simulink model "P6"  (R2019a)
settings: Solver=VariableStepAuto  StartTime=0.0  StopTime=20.0  RelTol=1e-3
undefined symbols (not defined in the file): P_reduced
settings Model: Creator=ADMIN  LastModifiedBy=ADMIN

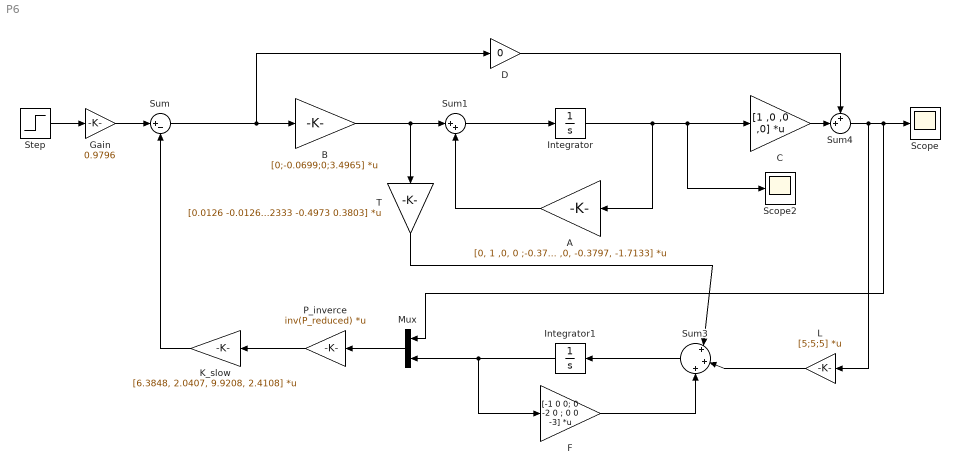
== system P6 ==
  A : Gain  Gain=[0, 1 ,0, 0 ;-0.378 ,0 ,7.0147 ,0.0343;0, 0, 0, 1; 18.9001 ,0, -0.3797, -1.7133]  Multiplication=Matrix(K*u) (u vector)
  B : Gain  Gain=[0;-0.0699;0;3.4965]  Multiplication=Matrix(K*u) (u vector)
  C : Gain  Gain=[1 ,0 ,0 ,0]  Multiplication=Matrix(K*u) (u vector)
  D : Gain  Gain=0
  F : Gain  Gain=[-1 0 0; 0 -2 0 ; 0 0 -3]  Multiplication=Matrix(K*u) (u vector)
  Gain : Gain  Gain=0.9796
  Integrator : Integrator
  Integrator1 : Integrator
  K_slow : Gain  Gain=[6.3848, 2.0407, 9.9208, 2.4108]  Multiplication=Matrix(K*u) (u vector)
  L : Gain  Gain=[5;5;5]  Multiplication=Matrix(K*u) (u vector)
  Mux : Mux  Inputs=2
  P_inverce : Gain  Gain=inv(P_reduced)  Multiplication=Matrix(K*u) (u vector)
  Scope : Scope
  Scope2 : Scope
  Step : Step  Time=0  After=0.1  SampleTime=0
  Sum : Sum  Inputs=|+-
  Sum1 : Sum  Inputs=|++
  Sum3 : Sum  Inputs=|+|+|+
  Sum4 : Sum  Inputs=++|
  T : Gain  Gain=[0.0126 -0.0126 0.1885 0.2636;-0.075 0.0375 -0.0796 0.2732; -0.6998 0.2333 -0.4973 0.3803]  Multiplication=Matrix(K*u) (u vector)
  wires:
  F/1 -> Sum3/3
  D/1 -> Sum4/1
  A/1 -> Sum1/2
  Integrator/1 -> A/1, C/1, Scope2/1
  C/1 -> Sum4/2
  Sum4/1 -> Mux/1, Scope/1, L/1
  B/1 -> Sum1/1, T/1
  Sum1/1 -> Integrator/1
  Gain/1 -> Sum/1
  Step/1 -> Gain/1
  K_slow/1 -> Sum/2
  Sum/1 -> B/1, D/1
  L/1 -> Sum3/2
  T/1 -> Sum3/1
  Sum3/1 -> Integrator1/1
  Integrator1/1 -> F/1, Mux/2
  P_inverce/1 -> K_slow/1
  Mux/1 -> P_inverce/1
